simulink model "ros_simulink_mssg_transmit"  (R2022b)
settings: Solver=VariableStepAuto  StartTime=0.0  StopTime=inf  RelTol=1e-3
values from neighbouring files (symbols this model uses):
  Pose = sim_out.Pose    [simulink_mobile_robot_sim.m]
undefined symbols (not defined in the file or in its folder): Linear
libraries: robotlib x3
settings Model: Creator=elmax  LastModifiedBy=elmax

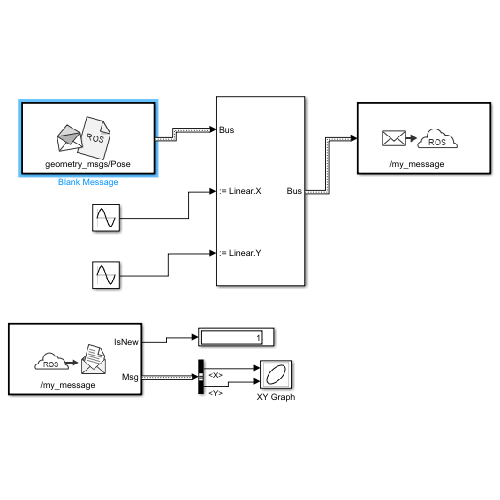
[thumbnail: Simulink's stored preview of the top-level diagram]
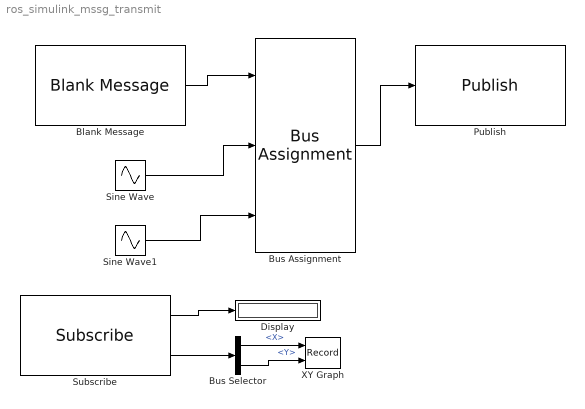
== system ros_simulink_mssg_transmit ==
  Blank Message : robotlib/Blank Message  messageClass=Message  entityType=geometry_msgs/Pose  messageType=geometry_msgs/Pose  SampleTime=inf  legacyBusStruct=off
      settings: LibrarySourceBlock=roslib/ROS/Blank Message
  Bus Assignment : BusAssignment  AssignedSignals=Linear.X,Linear.Y
  Bus Selector : BusSelector  OutputSignals=Linear.X,Linear.Y
  Display : Display
  Publish : robotlib/Publish  topicSource=Specify your own  topic=/my_message  messageType=geometry_msgs/Twist  legacyBusStruct=off  messageQueueLength=1
      settings: LibrarySourceBlock=roslib/ROS/Publish
  Sine Wave : Sin  SampleTime=0
  Sine Wave1 : Sin  Phase=pi/2  SampleTime=0
  Subscribe : robotlib/Subscribe  topicSource=Specify your own  topic=/my_message  messageType=geometry_msgs/Twist  SampleTime=-1  legacyBusStruct=off  messageQueueLength=1
      settings: LibrarySourceBlock=roslib/ROS/Subscribe
  XY Graph : Record  FileSettingsInternal="{\"entries\":[{\"content\":{\"excelSettings\":{\"content\":{},\"type\":\"Streamout.ExcelSettings\"}},\"type\":\"Streamout.FileSettingStorage\",\"uuid\":\"bb39adf9-836f-43bc-9339-2df6a82fc8ce\"}],\"packageUris\":[\"http://schema.mathworks.com/mf0/streamout_blocks/R2020a\"],\"version\":\"1.0\"}"  Layout=[1 1]  SignalsInternal="{\"entries\":[{\"content\":{\"signals\":[{\"content\":{\"blockPath\":[\"ros_simulink_mssg_transmit/XY Graph\"],\"channel\":[],\"dimensions\":[1],\"domain\":\"ros_simulink_mssg_transmit/XY Graph\",\"lineColor\":\"#a2142f\",\"plots\":[1],\"port\":1,\"sid\":[\"\"],\"signalID\":126,\"signalName\":\"<X>\"},\"type\":\"RecordBlkView.Signal\",\"uuid\":\"52dfb503-6d24-42ce-89cc-823181eba8d4\"},{\"content\":{\"blockPath\":[\"ros_simulink_mssg_transmit/XY Graph\"],\"channel\":[],\"dimensions\":[1],\"domain\":\"ros_simulink_mssg_transmit/XY Graph\",\"lineColor\":\"#139fff\",\"plots\":[1],\"port\":2,\"sid\":[\"\"],\"signalID\":130,\"signalName\":\"<Y>\"},\"type\":\"RecordBlkView.Signal\",\"uuid\":\"fd4e520d-c94b-4af6-9549-e91894780d6f\"}]},\"type\":\"RecordBlkView.InputSignals\",\"uuid\":\"75552957-9b7f-4f5e-bd4e-b53e49f28efb\"}],\"packageUris\":[\"http://schema.mathworks.com/mf0/streamout_blocks/R2020a\"],\"version\":\"1.0\"}"  VisualizationBindings="{\"xyplotplugin\":{\"info\":[{\"series\":[{\"bindingParametersList\":[{\"parameter\":\"X-Axis\",\"signalID\":126,\"signalName\":\"<X>\"},{\"parameter\":\"Y-Axis\",\"signalID\":130,\"signalName\":\"<Y>\"}],\"seriesID\":24794}],\"subplotID\":1}]}}"  CompatibilityTag=XY
  wires:
  Blank Message/1 -> Bus Assignment/1
  Bus Assignment/1 -> Publish/1
  Sine Wave/1 -> Bus Assignment/2
  Sine Wave1/1 -> Bus Assignment/3
  Subscribe/2 -> Bus Selector/1
  Bus Selector/1 -> XY Graph/1  "<X>"
  Bus Selector/2 -> XY Graph/2  "<Y>"
  Subscribe/1 -> Display/1
